simulink library "Spring_LeftRight_AsymmetricLinear"  (R2026a)
settings: Solver=VariableStepAuto
libraries: fl_lib x2, Spring_Linear x2
Description:
  | Component of Simscape Vehicle Templates Library
  | 
  | Copyright 2018-2026 The MathWorks, Inc.
settings Model: Creator=smiller  LastModifiedBy=smiller

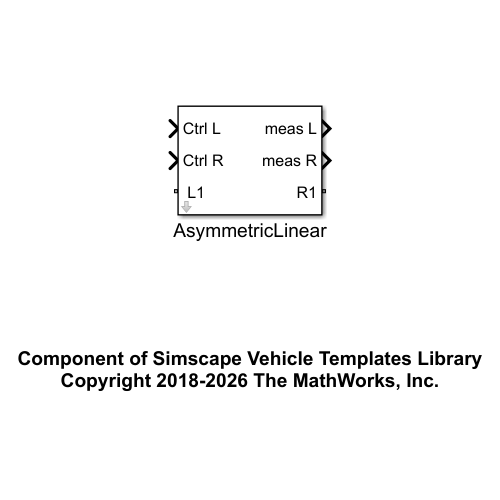
[thumbnail: Simulink's stored preview of the top-level diagram]
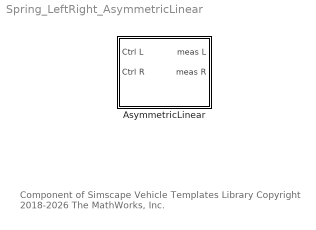
== system Spring_LeftRight_AsymmetricLinear ==
  note: Component of Simscape Vehicle Templates Library
      | Copyright 2018-2026 The MathWorks, Inc.
  AsymmetricLinear : Subsystem  VariantControl=Linear  mask(Asymmetric Linear Springs){}
      mask help: Springs with independent hardpoint parameterization for left and right sides. For spring connections in suspensions that may be asymmetric at design position, such as panhard rod suspensions.

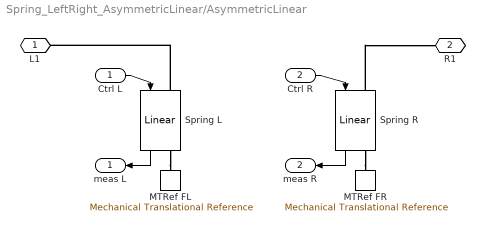
== system Spring_LeftRight_AsymmetricLinear/AsymmetricLinear ==
  Ctrl L : Inport
  Ctrl R : Inport  Port=2
  MTRef FL : fl_lib/Mechanical/Translational Elements/Mechanical Translational Reference
  MTRef FR : fl_lib/Mechanical/Translational Elements/Mechanical Translational Reference
  Spring L : Spring_Linear/Linear  VariantControl=Linear  spr_def0=Spring.xPreloadL.Value  spr_frc0=Spring.fPreloadL.Value  spr_k=Spring.K.Value  spr_hp_top=Spring.sTopL.Value  spr_hp_bot=Spring.sBottomL.Value
  Spring R : Spring_Linear/Linear  VariantControl=Linear  spr_def0=Spring.xPreloadR.Value  spr_frc0=Spring.fPreloadR.Value  spr_k=Spring.K.Value  spr_hp_top=Spring.sTopR.Value  spr_hp_bot=Spring.sBottomR.Value
  " L1" : PMIOPort  Side=Left
  R1 : PMIOPort  Port=2  Side=Right
  meas L : Outport  VectorParamsAs1DForOutWhenUnconnected=off
  meas R : Outport  Port=2  VectorParamsAs1DForOutWhenUnconnected=off
  wires:
  Ctrl L/1 -> Spring L/1
  Spring L/1 -> meas L/1
  Spring R/1 -> meas R/1
  Ctrl R/1 -> Spring R/1
  connections:
  Spring L/RConn1 -- MTRef FL/LConn1
  Spring R/RConn1 -- MTRef FR/LConn1
  Spring L/LConn1 -- " L1"/RConn1
  Spring R/LConn1 -- R1/RConn1
